simulink model "Kalman_tester"  (R2025b)
settings: Solver=VariableStepAuto  StartTime=0.0  StopTime=60  RelTol=1e-3
values from neighbouring files (symbols this model uses):
  dt = 0.01    [Data_Generation.m]
settings Model: Creator=Admin  LastModifiedBy=Admin

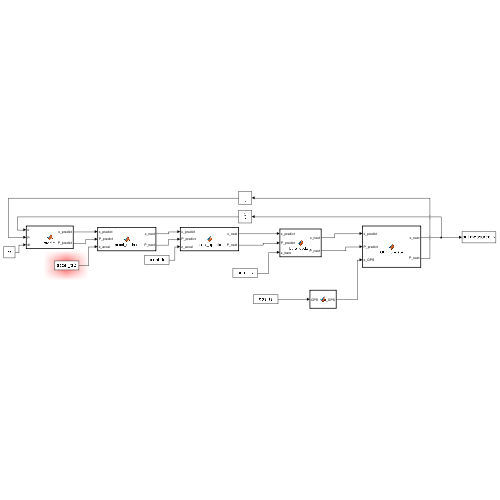
[thumbnail: Simulink's stored preview of the top-level diagram]
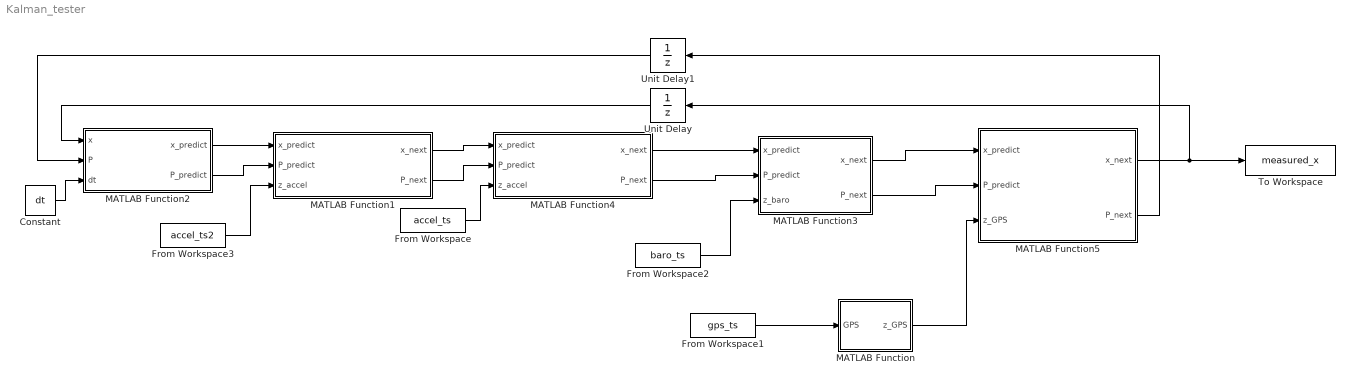
== system Kalman_tester ==
  Constant : Constant  Value=dt
  From Workspace : FromWorkspace  VariableName=accel_ts  SampleTime=dt
  From Workspace1 : FromWorkspace  VariableName=gps_ts  SampleTime=dt
  From Workspace2 : FromWorkspace  VariableName=baro_ts  SampleTime=dt
  From Workspace3 : FromWorkspace  VariableName=accel_ts2  SampleTime=dt
  MATLAB Function : MATLAB Function  TreatAsAtomicUnit=on
  MATLAB Function1 : MATLAB Function  TreatAsAtomicUnit=on
  MATLAB Function2 : MATLAB Function  TreatAsAtomicUnit=on
  MATLAB Function3 : MATLAB Function  TreatAsAtomicUnit=on
  MATLAB Function4 : MATLAB Function  TreatAsAtomicUnit=on
  MATLAB Function5 : MATLAB Function  TreatAsAtomicUnit=on
  To Workspace : ToWorkspace  VariableName=measured_x  SaveFormat=Timeseries  SampleTime=-1
  Unit Delay : UnitDelay  InitialCondition=zeros(9,1)  SampleTime=dt  HasFrameUpgradeWarning=on
  Unit Delay1 : UnitDelay  InitialCondition=zeros(9)  SampleTime=dt  HasFrameUpgradeWarning=on
  wires:
  MATLAB Function/1(z_GPS) -> MATLAB Function5/3(z_GPS)
  From Workspace/1 -> MATLAB Function4/3(z_accel)
  From Workspace1/1 -> MATLAB Function/1(GPS)
  MATLAB Function4/1(x_next) -> MATLAB Function3/1(x_predict)
  MATLAB Function4/2(P_next) -> MATLAB Function3/2(P_predict)
  From Workspace2/1 -> MATLAB Function3/3(z_baro)
  MATLAB Function3/1(x_next) -> MATLAB Function5/1(x_predict)
  MATLAB Function3/2(P_next) -> MATLAB Function5/2(P_predict)
  Constant/1 -> MATLAB Function2/3(dt)
  MATLAB Function5/1(x_next) -> Unit Delay/1, To Workspace/1
  MATLAB Function5/2(P_next) -> Unit Delay1/1
  Unit Delay/1 -> MATLAB Function2/1(x)
  Unit Delay1/1 -> MATLAB Function2/2(P)
  MATLAB Function1/1(x_next) -> MATLAB Function4/1(x_predict)
  MATLAB Function1/2(P_next) -> MATLAB Function4/2(P_predict)
  MATLAB Function2/1(x_predict) -> MATLAB Function1/1(x_predict)
  MATLAB Function2/2(P_predict) -> MATLAB Function1/2(P_predict)
  From Workspace3/1 -> MATLAB Function1/3(z_accel)

== matlab function Kalman_tester/MATLAB Function ==
  data: GPS input; z_GPS output
function z_GPS = z_calc(GPS)
%#codegen

GPS = GPS(:);  % enforce 6x1

lat0 = 51.507351;
lon0 = -0.127758;
h0   = 25;

% Tell Simulink these are interpreted MATLAB calls
coder.extrinsic('wgs84Ellipsoid','geodetic2ned');

spheroid = wgs84Ellipsoid("meter");

[pN, pE, pD] = geodetic2ned(GPS(1), GPS(2), GPS(3), lat0, lon0, h0, spheroid);

vN = GPS(4);
vE = GPS(5);
vD = GPS(6);

z_GPS = zeros(6,1);     % preallocate for Simulink sizing
z_GPS(:) = [pN; pE; pD; vN; vE; vD];
end

== matlab function Kalman_tester/MATLAB Function1 ==
  data: x_predict input; x_next output; P_predict input; z_accel input; P_next output
function [x_next, P_next] = accel_update(x_predict, P_predict, z_accel)

sigma_accel = 0.05;
R = (sigma_accel^2) * eye(3);   % 3x3

I = eye(3);
Z = zeros(3);

H = [Z, Z, I];
S   = H * P_predict * H' + R;
K_k = (P_predict * H') / S;

x_next = x_predict + K_k * (z_accel - H * x_predict);
P_next = (eye(9) - K_k * H) * P_predict;

end

== matlab function Kalman_tester/MATLAB Function2 ==
  data: x input; x_predict output; P input; P_predict output; dt input
function [x_predict, P_predict] = predict(x, P, dt)

sigma_jerk = 0.5;       % m/s^3  (tune)
qj = sigma_jerk^2;
I = eye(3);
Z = zeros(3);

Q_sub = qj*[dt^6/9, dt^5/6, dt^4/3;
            dt^5/6, dt^4/4, dt^3/2;
            dt^4/3, dt^3/2, dt^2];

Q = kron(Q_sub, eye(3));

A = [I,  dt*I,  (0.5*dt^2)*I;
     Z,    I,     dt*I      ;
     Z,    Z,       I       ];
x_predict = A * x;
P_predict = A * P * A' + Q;

end

== matlab function Kalman_tester/MATLAB Function3 ==
  data: x_predict input; x_next output; P_predict input; z_baro input; P_next output
function [x_next, P_next] = baro_update(x_predict, P_predict, z_baro)

sigma_baro = 1.0;   % meters

R = sigma_baro^2;


H = [0, 0, 1, zeros(1, 6)];
S   = H * P_predict * H' + R;
K_k = (P_predict * H') / S;

x_next = x_predict + K_k * (z_baro - H * x_predict);
P_next = (eye(9) - K_k * H) * P_predict;

end

== matlab function Kalman_tester/MATLAB Function4 ==
  data: x_predict input; x_next output; P_predict input; z_accel input; P_next output
function [x_next, P_next] = accel_update(x_predict, P_predict, z_accel)

sigma_accel = 0.05;
R = (sigma_accel^2) * eye(3);   % 3x3

I = eye(3);
Z = zeros(3);

H = [Z, Z, I];
S   = H * P_predict * H' + R;
K_k = (P_predict * H') / S;

x_next = x_predict + K_k * (z_accel - H * x_predict);
P_next = (eye(9) - K_k * H) * P_predict;

end

== matlab function Kalman_tester/MATLAB Function5 ==
  data: x_predict input; x_next output; P_predict input; z_GPS input; P_next output
function [x_next, P_next] = GPS_update(x_predict, P_predict, z_GPS)

x_predict = x_predict(:);
z_GPS = z_GPS(:);

sigma_gps_pos = 1.5;
sigma_gps_vel = 0.1;

R = diag([ ...
    (sigma_gps_pos^2)*ones(3,1); ...
    (sigma_gps_vel^2)*ones(3,1) ...
]);  % 6x6

I = eye(3);
Z = zeros(3);

H = [I, Z, Z;
     Z, I, Z];
S   = H * P_predict * H' + R;
K_k = (P_predict * H') / S;

x_next = x_predict + K_k * (z_GPS - H * x_predict);
P_next = (eye(9) - K_k * H) * P_predict;

end
